simulink model "sim_explicit_MPC_N"  (R2017b)
settings: Solver=VariableStepAuto  StartTime=0.0  StopTime=50  RelTol=1e-3
values from neighbouring files (symbols this model uses):
  g = 9.81    [init_sim.m]
  m = 0.03    [init_sim.m]
  mpc_phi = str2func(c)    [get_sim_data_mpc_phi.m]    (also in get_sim_data_mpc_y.m = @(x) quad_mpc_tree_phi(x); get_sim_data_mpc_z.m = @(x) quad_mpc_tree_phi(x))
  mpc_y = @(x) quad_mpc_tree_y(x)    [get_sim_data_mpc_phi.m]    (also in get_sim_data_mpc_y.m = str2func(c); get_sim_data_mpc_z.m)
  mpc_z = @(x) quad_mpc_tree_z(x)    [get_sim_data_mpc_phi.m]    (also in get_sim_data_mpc_y.m; get_sim_data_mpc_z.m = str2func(c))
  Ts = 1e-2    (= 0.01)    [init_sim.m]
  u_max = [f_max; tau_max]    [init_sim.m]
  u_min = [f_min; tau_min]    [init_sim.m]
  x0 = zeros(6,1)    [get_sim_data.m]    (also in get_sim_data_mpc_phi.m; get_sim_data_mpc_y.m; get_sim_data_mpc_z.m; init_sim.m = 0.9*[InvSet_y.V(i,1)'; InvSet_z.V(j,1)'; InvSet_phi.V(k,1)';)
  x_max = [y_max;z_max;angle_max;vy_max;vz_max;arate_max]    [init_sim.m]
  x_min = [y_min;z_min;angle_min;vy_min;vz_min;arate_min]    [init_sim.m]
undefined symbols (not defined in the file or in its folder): uavPlanarNonlin
settings Model: Creator=zboucek  LastModifiedBy=zdenek

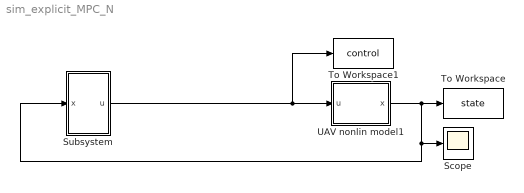
== system sim_explicit_MPC_N ==
  Scope : Scope
  Subsystem : Subsystem
  To Workspace : ToWorkspace  VariableName=state  SaveFormat=Structure With Time  SampleTime=Ts
  To Workspace1 : ToWorkspace  VariableName=control  SaveFormat=Structure With Time  SampleTime=Ts
  UAV nonlin model1 : Subsystem
  wires:
  UAV nonlin model1/1(x) -> Subsystem/1(x), Scope/1, To Workspace/1
  Subsystem/1(u) -> To Workspace1/1, UAV nonlin model1/1(u)

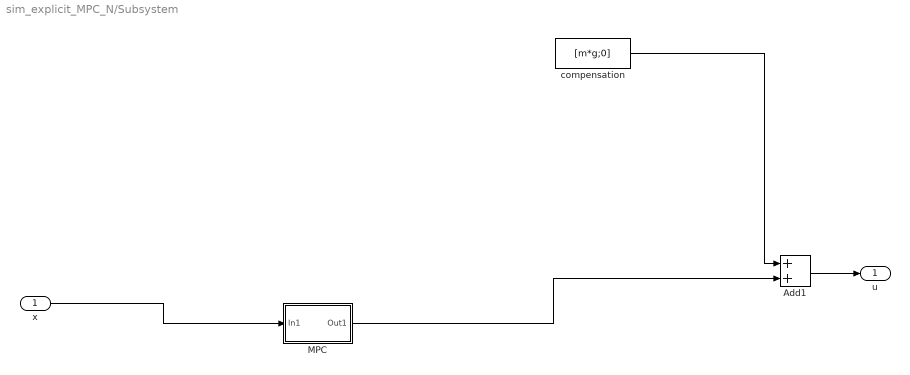
== system sim_explicit_MPC_N/Subsystem ==
  x : Inport
  Add1 : Sum
  MPC : Subsystem
  compensation : Constant  Value=[m*g;0]
  u : Outport
  wires:
  Add1/1 -> u/1
  compensation/1 -> Add1/1
  x/1 -> MPC/1(In1)
  MPC/1(Out1) -> Add1/2

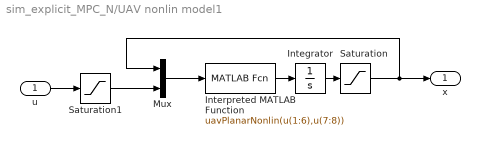
== system sim_explicit_MPC_N/UAV nonlin model1 ==
  u : Inport
  Integrator : Integrator  InitialCondition=x0
  Interpreted MATLAB Function : MATLABFcn  MATLABFcn=uavPlanarNonlin(u(1:6),u(7:8))  OutputDimensions=6
  Mux : Mux  Inputs=2
  Saturation : Saturate  UpperLimit=x_max  LowerLimit=x_min
  Saturation1 : Saturate  UpperLimit=u_max  LowerLimit=u_min
  x : Outport
  wires:
  Mux/1 -> Interpreted MATLAB Function/1
  Interpreted MATLAB Function/1 -> Integrator/1
  u/1 -> Saturation1/1
  Integrator/1 -> Saturation/1
  Saturation/1 -> Mux/1, x/1
  Saturation1/1 -> Mux/2

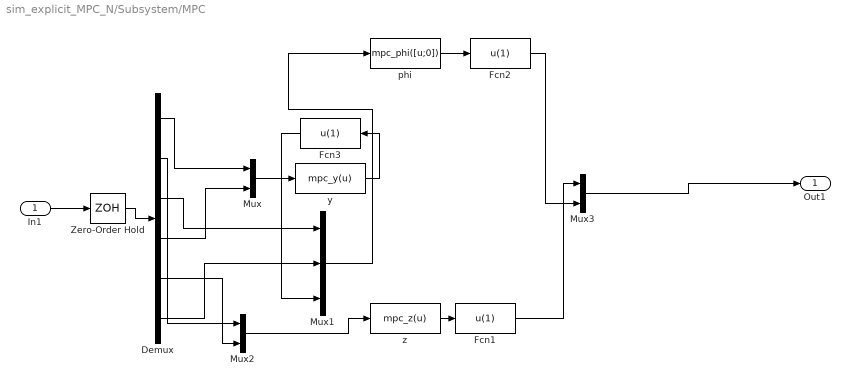
== system sim_explicit_MPC_N/Subsystem/MPC ==
  In1 : Inport
  Demux : Demux  Outputs=6
  Fcn1 : Fcn  Expr=u(1)
  Fcn2 : Fcn  Expr=u(1)
  Fcn3 : Fcn  Expr=u(1)
  Mux : Mux  Inputs=2
  Mux1 : Mux  Inputs=3
  Mux2 : Mux  Inputs=2
  Mux3 : Mux  Inputs=2
  Zero-Order Hold : ZeroOrderHold  SampleTime=Ts
  phi : MATLABFcn  MATLABFcn=mpc_phi([u;0])
  y : MATLABFcn  MATLABFcn=mpc_y(u)
  z : MATLABFcn  MATLABFcn=mpc_z(u)
  Out1 : Outport
  wires:
  Demux/4 -> Mux/2
  Mux2/1 -> z/1
  Demux/1 -> Mux/1
  Mux/1 -> y/1
  Demux/3 -> Mux1/1
  y/1 -> Fcn3/1
  Demux/2 -> Mux2/1
  Mux3/1 -> Out1/1
  In1/1 -> Zero-Order Hold/1
  Zero-Order Hold/1 -> Demux/1
  phi/1 -> Fcn2/1
  z/1 -> Fcn1/1
  Fcn1/1 -> Mux3/1
  Fcn2/1 -> Mux3/2
  Mux1/1 -> phi/1
  Fcn3/1 -> Mux1/3
  Demux/6 -> Mux1/2
  Demux/5 -> Mux2/2
